simulink model "Base_isolated_structure_LSTM"  (R2024a)
settings: Solver=ode4  StartTime=0.0  StopTime=tend  FixedStep=dt  RelTol=1e-3
values from neighbouring files (symbols this model uses):
  As = [zeros(24,24) eye(24) zeros(24,6);MK-R*m_RK MC-R*m_RC zeros(24,6);zeros(3,51) eye(3);m_RK m_RC zeros(3,6)]    [Base_isolated_structure_main.m]
  Bs = [zeros(24,6);zeros(24,3) R/m;zeros(3,6);-eye(3) -inv(m)]    [Base_isolated_structure_main.m]
  Cs = eye(54)    [Base_isolated_structure_main.m]
  Ds = zeros(54,6)    [Base_isolated_structure_main.m]
  dt = 0.002    [BLWN_training_data_prep.m]    (also in Base_isolated_structure_main.m; Inter_story_damped_structure_MBW_main.m; Inter_story_damped_structure_MFD_main.m)
  Fscale = 80    [Base_isolated_structure_main.m]
  MBW_locs = All_locs(32:61,2:3)    [Base_isolated_structure_plan.m]
  MFD_locs = All_locs(1:31,2:3)    [Base_isolated_structure_plan.m]
  Reduce2 = zeros(3,54);Reduce2(:,49:51)=eye(3)    [Base_isolated_structure_main.m]
  uscale = 0.1    [Base_isolated_structure_main.m]
libraries: deeplib x2
settings Model: Creator=tujia  LastModifiedBy=li292
settings SolverCC: AlgebraicLoopSolver=TrustRegion
settings DataIOCC: ReturnWorkspaceOutputs=off
settings OptimizationCC: LifeSpan=inf
settings DebuggingCC: SigSpecEnsureSampleTimeMsg=none  UnconnectedInputMsg=warning  UnconnectedOutputMsg=warning  UnconnectedLineMsg=warning  ArithmeticOperatorsInVariantConditions=warning
settings ModelReferenceCC: EnableRefExpFcnMdlSchedulingChecks=on
settings SFSimCC: SimUseLocalCustomCode=off  CustomCodeUndefinedFunction=UseInterfaceOnly
settings RTWCC: RTWUseLocalCustomCode=off  GPUComputeCapability=3.5
settings CodeAppCC: StateflowObjectComments=on

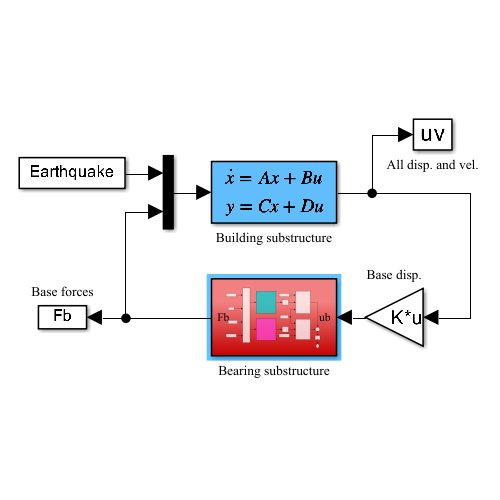
[thumbnail: Simulink's stored preview of the top-level diagram]
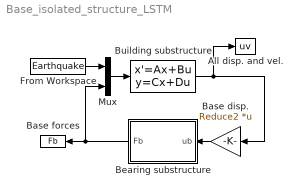
== system Base_isolated_structure_LSTM ==
  All disp. and vel. : ToWorkspace  VariableName=uv  SampleTime=dt
      settings: Save2DSignal=2-D array (concatenate along first dimension)
  Base disp. : Gain  Gain=Reduce2  Multiplication=Matrix(K*u)
  Base forces : ToWorkspace  VariableName=Fb  SampleTime=dt
      settings: Save2DSignal=2-D array (concatenate along first dimension)
  Bearing substructure : Subsystem
  Building substructure : StateSpace  A=As  B=Bs  C=Cs  D=Ds  InitialCondition=zeros(54,1)
  From Workspace : FromWorkspace  VariableName=Earthquake
  Mux : Mux  Inputs=2
  wires:
  Base disp./1 -> Bearing substructure/1(ub)
  Mux/1 -> Building substructure/1
  Building substructure/1 -> Base disp./1, All disp. and vel./1
  From Workspace/1 -> Mux/1
  Bearing substructure/1(Fb) -> Base forces/1, Mux/2

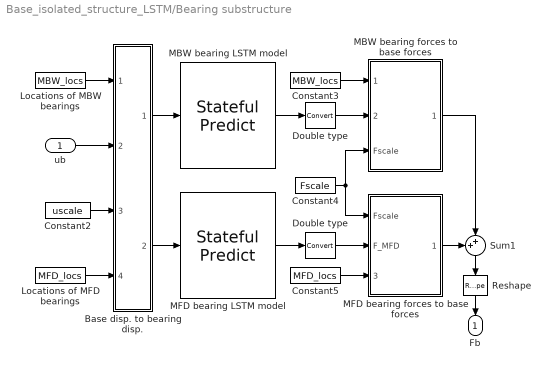
== system Base_isolated_structure_LSTM/Bearing substructure ==
  ub : Inport
  " Double type " : DataTypeConversion  SaturateOnIntegerOverflow=off  RndMeth=Floor
  Base disp. to bearing disp. : MATLAB Function  TreatAsAtomicUnit=on
  Constant2 : Constant  Value=uscale
  Constant3 : Constant  Value=MBW_locs
  Constant4 : Constant  Value=Fscale
  Constant5 : Constant  Value=MFD_locs
  Double type : DataTypeConversion  SaturateOnIntegerOverflow=off  RndMeth=Floor
  Locations of MBW bearings : Constant  Value=MBW_locs
  Locations of MFD bearings : Constant  Value=MFD_locs
  MBW bearing LSTM model : deeplib/Stateful Predict  Network=Network from MAT-file  NetworkFunction=untitled  NetworkFilePath=MBW_Simulink.mat  InputDataFormats={ 'sequenceinput', 'TBC' }  SampleTime=dt  ForceInterpretedSim=off  EnableDLNetwork=on  LastKnownNetworkFilePath=''  LastKnownNetworkTimeStamp=''
  MBW bearing forces to base forces : MATLAB Function  TreatAsAtomicUnit=on
  MFD bearing LSTM model : deeplib/Stateful Predict  Network=Network from MAT-file  NetworkFunction=untitled  NetworkFilePath=MFD_Simulink.mat  InputDataFormats={ 'sequenceinput', 'TBC' }  SampleTime=dt  ForceInterpretedSim=off  EnableDLNetwork=on  LastKnownNetworkFilePath=''  LastKnownNetworkTimeStamp=''
  MFD bearing forces to base forces : MATLAB Function  TreatAsAtomicUnit=on
  Reshape : Reshape
  Sum1 : Sum  Inputs=++|
  Fb : Outport
  wires:
  Locations of MBW bearings/1 -> Base disp. to bearing disp./1(MBW_locs)
  ub/1 -> Base disp. to bearing disp./2(ub)
  Locations of MFD bearings/1 -> Base disp. to bearing disp./4(MFD_locs)
  Constant3/1 -> MBW bearing forces to base forces/1(MBW_locs)
  Constant5/1 -> MFD bearing forces to base forces/3(MFD_locs)
  Sum1/1 -> Reshape/1
  MBW bearing LSTM model/1 -> Double type/1
  Base disp. to bearing disp./1(MBW_u) -> MBW bearing LSTM model/1
  Double type/1 -> MBW bearing forces to base forces/2(F_MBW)
  " Double type "/1 -> MFD bearing forces to base forces/2(F_MFD)
  MFD bearing LSTM model/1 -> " Double type "/1
  Base disp. to bearing disp./2(MFD_u) -> MFD bearing LSTM model/1
  Constant2/1 -> Base disp. to bearing disp./3(uscale)
  Constant4/1 -> MBW bearing forces to base forces/3(Fscale), MFD bearing forces to base forces/1(Fscale)
  MFD bearing forces to base forces/1(Fb_MFD) -> Sum1/1
  MBW bearing forces to base forces/1(Fb_MBW) -> Sum1/2
  Reshape/1 -> Fb/1

== matlab function Base_isolated_structure_LSTM/Bearing substructure/Base disp. to bearing disp. ==
  data: MBW_locs input; ub input; uscale input; MBW_u output; MFD_locs input; MFD_u output
function [MBW_u,MFD_u] = fcn(MBW_locs,ub,uscale, MFD_locs)
BW_u1=ub(1)-ub(3)*MBW_locs(:,2)';
BW_u2=ub(2)+ub(3)*MBW_locs(:,1)';
MBW_u = [BW_u1 BW_u2]*uscale*1000;

FDZ_u1=ub(1)-ub(3)*MFD_locs(:,2)';
FDZ_u2=ub(2)+ub(3)*MFD_locs(:,1)';
MFD_u = [FDZ_u1 FDZ_u2]*uscale*1000;

== matlab function Base_isolated_structure_LSTM/Bearing substructure/MBW bearing forces to base forces ==
  data: MBW_locs input; F_MBW input; Fb_MBW output; Fscale input
function Fb_MBW = fcn(MBW_locs,F_MBW,Fscale)
Fx=sum(F_MBW(1:30));
Fy=sum(F_MBW(30+1:end));
Fr=-sum(F_MBW(1:30).*MBW_locs(:,2)')+sum(F_MBW(30+1:end).*MBW_locs(:,1)');
Fb_MBW=[Fx;Fy;Fr]*Fscale;

== matlab function Base_isolated_structure_LSTM/Bearing substructure/MFD bearing forces to base forces ==
  data: Fscale input; F_MFD input; MFD_locs input; Fb_MFD output
function Fb_MFD = fcn(Fscale,F_MFD,MFD_locs)
Fx=sum(F_MFD(1:31));
Fy=sum(F_MFD(31+1:end));
Fr=-sum(F_MFD(1:31).*MFD_locs(:,2)')+sum(F_MFD(31+1:end).*MFD_locs(:,1)');
Fb_MFD=[Fx;Fy;Fr]*Fscale;
